simulink model "detumbling"  (R2023b)
settings: Solver=VariableStepAuto  StartTime=0.0  StopTime=10.0  RelTol=1e-3
values from neighbouring files (symbols this model uses):
  ARW = deg2rad(0.10)    [main_group24.m]
  Cd = 2.2    [main_group24.m]
  GyroSampleRate = 10    [main_group24.m]
  Ix = J(1,1)    [Air_Drag_script.m]    (also in data_mass.m = 0.0755003333333; main.m = 0.057749855; main_group24.m = 0.0755003333333)
  Iy = J(2,2)    [Air_Drag_script.m]    (also in data_mass.m = 0.0755003333333; main.m = 0.04143542; main_group24.m = 0.0755003333333)
  Iz = J(3,3)    [Air_Drag_script.m]    (also in data_mass.m = 0.055; main.m = 0.024624309; main_group24.m = 0.055)
  J = diag([100.9 25.1 91.6])*1e-2    [Air_Drag_script.m]
  MMnoise = 15e-9*[1; 1; 1]    [main_group24.m]
  MMSampleRate = 1    [main_group24.m]
  P = Fe/c    (= 4.52980041279e-06)    [main_group24.m]
  rho_air = 1.65e-13    [Air_Drag_script.m]    (also in main_group24.m = 6.967e-13)
  rho_d_body = 0.1*2/3    (= 0.0666666666667)    [main_group24.m]
  rho_d_sp = 0.1*2/3    (= 0.0666666666667)    [main_group24.m]
  rho_s_body = 0.5    [main_group24.m]
  rho_s_sp = 0.1    [main_group24.m]
  RRW = deg2rad(0.3)    [main_group24.m]
undefined symbols (not defined in the file or in its folder): invJ, omega_0b, pan1, pan2, s1, s2, s3, s4, s5, s6, v_rel
libraries: vrlib x21, sharedutil x2
settings Model: Creator=hp  LastModifiedBy=hp

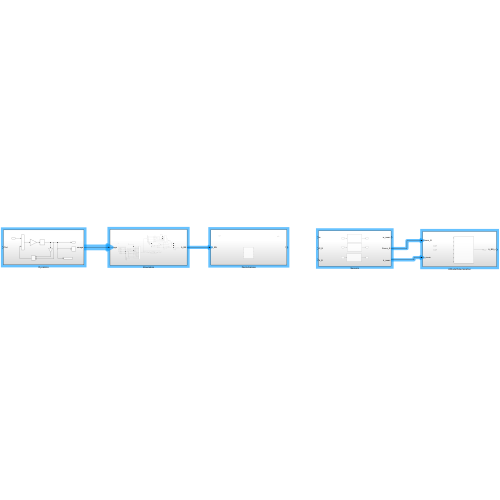
[thumbnail: Simulink's stored preview of the top-level diagram]
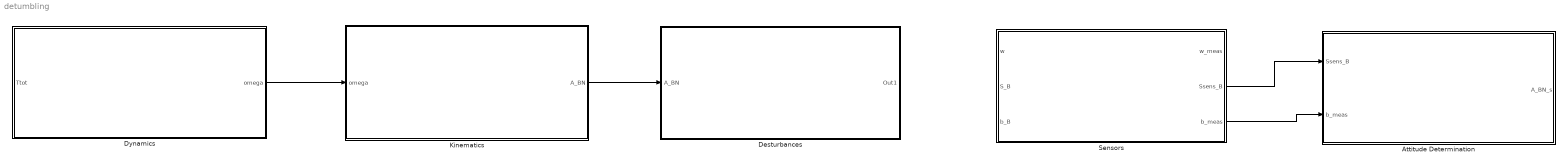
== system detumbling ==
  Attitude Determination : Subsystem
  Desturbances : Subsystem
  Dynamics : Subsystem
  Kinematics : Subsystem
  Sensors : Subsystem
  wires:
  Sensors/3(b_meas) -> Attitude Determination/2(b_meas)
  Kinematics/1(A_BN) -> Desturbances/1(A_BN)
  Sensors/2(Ssens_B) -> Attitude Determination/1(Ssens_B)
  Dynamics/1(omega) -> Kinematics/1(omega)

== system detumbling/Attitude Determination ==
  Ssens_B : Inport
  b_meas : Inport  Port=2
  Attitude Determination : MATLAB Function  TreatAsAtomicUnit=on
  A_BN_s : Outport
  wires:
  Attitude Determination/1(A_BN_s) -> A_BN_s/1  "A_BN_s"

== system detumbling/Desturbances ==
  A_BN : Inport
  Disturbance : Subsystem
  Out1 : Outport

== system detumbling/Dynamics ==
  note: omega
  Ttot : Inport
  Add : Sum
  Cross Product : vrlib/Utilities/Cross Product
  Gain : Gain  Gain=invJ  Multiplication=Matrix(K*u)
  Gain1 : Gain  Gain=J  Multiplication=Matrix(K*u)
  Integrator3 : Integrator  InitialCondition=omega_0b  AbsoluteTolerance=10^-7
  Scope : Scope
  To Workspace : ToWorkspace  VariableName=det  SaveFormat=Timeseries  SampleTime=-1
  omega : Outport
  wires:
  Gain1/1 -> Cross Product/1
  Ttot/1 -> Add/1
  Cross Product/1 -> Add/2
  Integrator3/1 -> To Workspace/1, Scope/1, omega/1, Cross Product/2, Gain1/1
  Gain/1 -> Integrator3/1
  Add/1 -> Gain/1

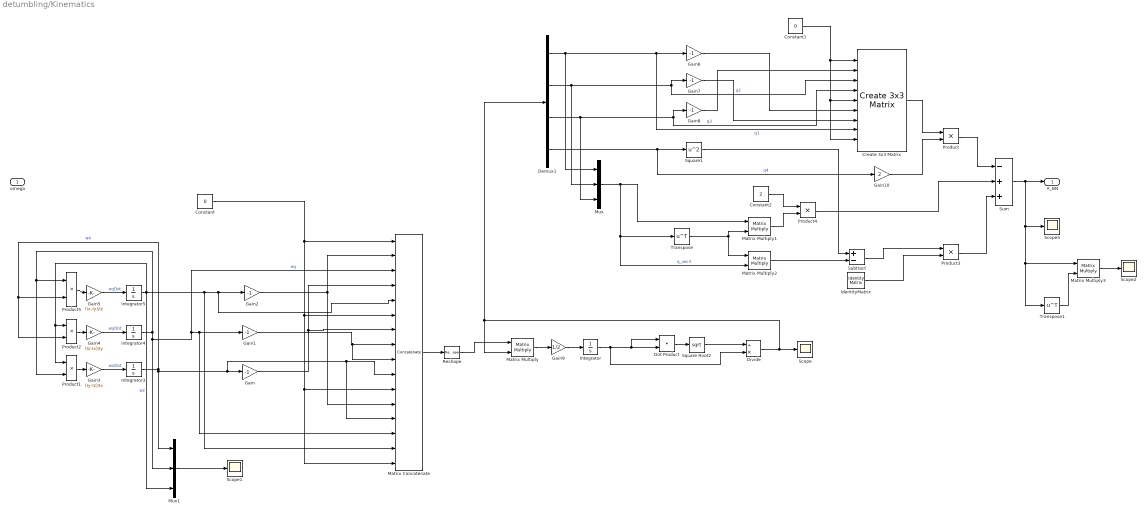
== system detumbling/Kinematics ==
  omega : Inport
  Constant : Constant  Value=0
  Constant1 : Constant  Value=0
  Constant2 : Constant  Value=2
  Create 3x3 Matrix : sharedutil/Create 3x3 Matrix  aMode=aMode
      settings: LibrarySourceBlock=aerolibutil/Create 3x3 Matrix
  Demux1 : Demux
  Divide : Product  Inputs=/*
  Dot Product : DotProduct  OutDataTypeStr=Inherit: Inherit via internal rule
  Gain{,1..2,6..8} (6 alike) : Gain  Gain=-1
  Gain10 : Gain  Gain=2
  Gain3 : Gain  Gain=(Iy-Iz)/Ix
  Gain4 : Gain  Gain=(Iz-Ix)/Iy
  Gain5 : Gain  Gain=(Ix-Iy)/Iz
  Gain9 : Gain  Gain=1/2
  IdentityMatrix : IdentityMatrix  OutputDimensions=3
  Integrator : Integrator  InitialCondition=[0 0 0 1]
  Integrator3 : Integrator  InitialCondition=omega_0b(1)
  Integrator4 : Integrator  InitialCondition=omega_0b(2)
  Integrator5 : Integrator  InitialCondition=omega_0b(3)
  Matrix Concatenate : Concatenate  NumInputs=16  Mode=Multidimensional array  ConcatenateDimension=2
  Matrix Multiply{,1..3} (4 alike) : Product  Multiplication=Matrix(*)
  Mux : Mux  Inputs=3
  Mux1 : Mux  Inputs=3
  Product{,1..5} (6 alike) : Product
  Reshape : Reshape  OutputDimensionality=Customize  OutputDimensions=[4,4]
  Scope{,1..2,5} (4 alike) : Scope
  Square Root2 : Sqrt
  Square1 : Math  Operator=square
  Subtract : Sum  Inputs=+-
  Sum : Sum  Inputs=-++
  Transpose : Math  Operator=transpose
  Transpose1 : Math  Operator=transpose
  A_BN : Outport
  wires:
  Matrix Multiply/1 -> Gain9/1
  Square Root2/1 -> Divide/1
  Product1/1 -> Gain3/1
  Gain1/1 -> Matrix Concatenate/9, Matrix Concatenate/8
  Product5/1 -> Gain5/1
  Constant/1 -> Matrix Concatenate/16, Matrix Concatenate/11, Matrix Concatenate/6, Matrix Concatenate/1
  Gain3/1 -> Integrator3/1  "wxDot"
  Gain/1 -> Matrix Concatenate/7, Matrix Concatenate/4
  Integrator/1 -> Dot Product/1, Dot Product/2, Divide/2
  Matrix Concatenate/1 -> Reshape/1
  Integrator5/1 -> Mux1/3, Matrix Concatenate/15, Matrix Concatenate/5, Gain2/1, Product1/1, Product2/1  "wz"
  Gain4/1 -> Integrator4/1  "wyDot"
  Gain2/1 -> Matrix Concatenate/12, Matrix Concatenate/2
  Gain5/1 -> Integrator5/1  "wzDot"
  Integrator4/1 -> Matrix Concatenate/3, Matrix Concatenate/14, Gain1/1, Mux1/2, Product1/2, Product5/1  "wy"
  Integrator3/1 -> Matrix Concatenate/13, Matrix Concatenate/10, Gain/1, Mux1/1, Product2/2, Product5/2  "wx"
  Product2/1 -> Gain4/1
  Constant1/1 -> Create 3x3 Matrix/5, Create 3x3 Matrix/9, Create 3x3 Matrix/1
  Demux1/1 -> Mux/1, Gain6/1, Create 3x3 Matrix/8  "q1"
  Demux1/2 -> Mux/2, Gain7/1, Create 3x3 Matrix/3  "q2"
  Demux1/4 -> Gain10/1, Square1/1  "q4"
  Gain8/1 -> Create 3x3 Matrix/2
  Gain6/1 -> Create 3x3 Matrix/6
  Gain7/1 -> Create 3x3 Matrix/7
  Transpose/1 -> Matrix Multiply1/2, Matrix Multiply2/1
  Gain10/1 -> Product/2
  Create 3x3 Matrix/1 -> Product/1
  Square1/1 -> Subtract/1
  Matrix Multiply2/1 -> Subtract/2
  Divide/1 -> Scope/1, Demux1/1, Matrix Multiply/2
  Subtract/1 -> Product3/1
  IdentityMatrix/1 -> Product3/2
  Product/1 -> Sum/1
  Product3/1 -> Sum/3
  Constant2/1 -> Product4/1
  Matrix Multiply1/1 -> Product4/2
  Product4/1 -> Sum/2
  Demux1/3 -> Mux/3, Gain8/1, Create 3x3 Matrix/4  "q3"
  Mux/1 -> Matrix Multiply1/1, Transpose/1, Matrix Multiply2/2  "q_vec3"
  Mux1/1 -> Scope1/1
  Sum/1 -> Transpose1/1, Matrix Multiply3/1, Scope5/1, A_BN/1
  Transpose1/1 -> Matrix Multiply3/2
  Matrix Multiply3/1 -> Scope2/1
  Dot Product/1 -> Square Root2/1
  Reshape/1 -> Matrix Multiply/1
  Gain9/1 -> Integrator/1

== system detumbling/Sensors ==
  w : Inport
  S_B : Inport  Port=2
  b_B : Inport  Port=3
  Gyroscope : Subsystem
  Magnetometer : Subsystem
  Sun Sensor : Subsystem
  w_meas : Outport
  Ssens_B : Outport  Port=2
  b_meas : Outport  Port=3
  wires:
  w/1 -> Gyroscope/1(w)
  Gyroscope/1(w_meas) -> w_meas/1
  Sun Sensor/1(Ssens_B) -> Ssens_B/1
  S_B/1 -> Sun Sensor/1(S_B)
  b_B/1 -> Magnetometer/1(b_B)
  Magnetometer/1(MM_meas) -> b_meas/1

== system detumbling/Desturbances/Disturbance ==
  r_s_B : Inport
  v_rel_B : Inport  Port=2
  In4 : Inport  Port=3
  Air Drag : Subsystem
  Gravity Gradient : Subsystem
  Magnetic Field : Subsystem
  Solar Rsdiation Pressure : Subsystem
  Tsrp : Outport
  Tair : Outport  Port=2
  Out3 : Outport  Port=3
  Out4 : Outport  Port=4
  wires:
  r_s_B/1 -> Solar Rsdiation Pressure/1(r_s_B)
  In4/1 -> Magnetic Field/1(In1)
  Air Drag/1(Tair) -> Tair/1
  v_rel_B/1 -> Air Drag/1(v_rel_B)
  Magnetic Field/1(Out1) -> Out4/1
  Solar Rsdiation Pressure/1(Tsrp) -> Tsrp/1
  Gravity Gradient/1(Out1) -> Out3/1

== system detumbling/Sensors/Gyroscope ==
  note: w_BN_measured = G(w_B) A_eps w_BN + n + b
  w : Inport
  ARW : RandomNumber  Variance=(deg2rad(ARW)/sqrt(3600)/sqrt(1/GyroSampleRate))^2*[1;1;1]  SampleTime=1/GyroSampleRate
  Integrator : Integrator
  RRW : RandomNumber  Variance=(deg2rad(RRW)/3600/sqrt(1/GyroSampleRate))^2* [1;1;1]  SampleTime=1/GyroSampleRate
  Sensor Sampling frequency : ZeroOrderHold  SampleTime=-1
  Sum : Sum  Inputs=+++
  w_meas : Outport
  wires:
  RRW/1 -> Integrator/1  "b_dot"
  ARW/1 -> Sum/2  "n"
  Integrator/1 -> Sum/3  "b"
  w/1 -> Sensor Sampling frequency/1
  Sum/1 -> w_meas/1
  Sensor Sampling frequency/1 -> Sum/1

== system detumbling/Sensors/Magnetometer ==
  b_B : Inport
  Constant : Constant  Value=MMnoise
  MatrixMultiply : Product  Multiplication=Matrix(*)
  Subsystem : Subsystem
  Sum : Sum
  MM_meas : Outport
  wires:
  Constant/1 -> Sum/2
  b_B/1 -> Sum/1  "b_B"
  Subsystem/1(A_epsMM) -> MatrixMultiply/1
  Sum/1 -> MatrixMultiply/2
  MatrixMultiply/1 -> MM_meas/1

== system detumbling/Sensors/Sun Sensor ==
  S_B : Inport
  Matrix Multiply1 : Product  Multiplication=Matrix(*)
  Subsystem : Subsystem
  Ssens_B : Outport
  wires:
  S_B/1 -> Matrix Multiply1/2
  Subsystem/1(A_eps) -> Matrix Multiply1/1  "A_eps"
  Matrix Multiply1/1 -> Ssens_B/1

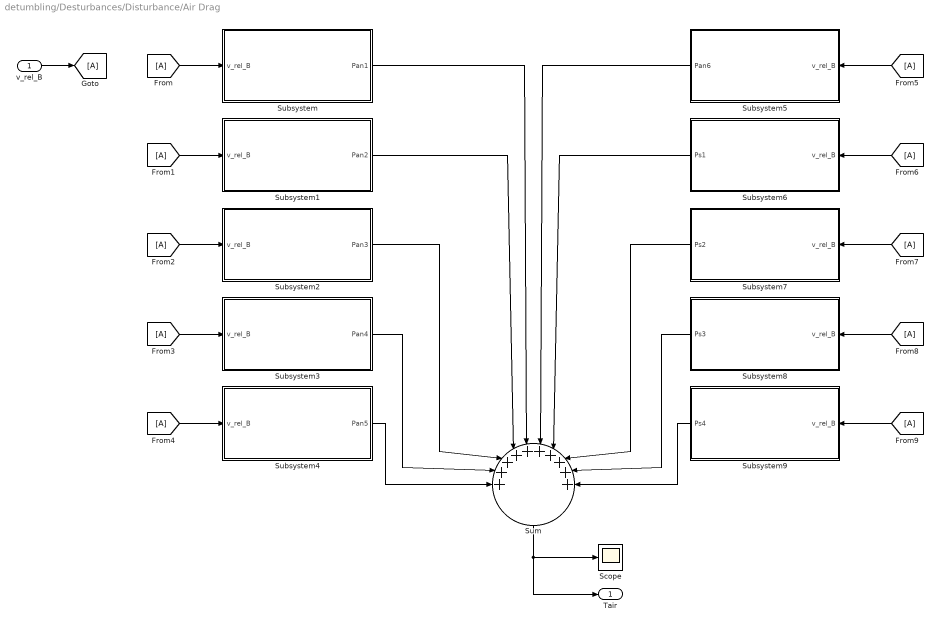
== system detumbling/Desturbances/Disturbance/Air Drag ==
  v_rel_B : Inport
  From{,1..9} (10 alike) : From
  Goto : Goto
  Scope : Scope
  Subsystem : Subsystem
  Subsystem1 : Subsystem
  Subsystem2 : Subsystem
  Subsystem3 : Subsystem
  Subsystem4 : Subsystem
  Subsystem5 : Subsystem
  Subsystem6 : Subsystem
  Subsystem7 : Subsystem
  Subsystem8 : Subsystem
  Subsystem9 : Subsystem
  Sum : Sum  Inputs=++++++++++
  Tair : Outport
  wires:
  Sum/1 -> Scope/1, Tair/1
  v_rel_B/1 -> Goto/1
  From5/1 -> Subsystem5/1(v_rel_B)
  From6/1 -> Subsystem6/1(v_rel_B)
  From7/1 -> Subsystem7/1(v_rel_B)
  From8/1 -> Subsystem8/1(v_rel_B)
  From9/1 -> Subsystem9/1(v_rel_B)
  From4/1 -> Subsystem4/1(v_rel_B)
  From3/1 -> Subsystem3/1(v_rel_B)
  From2/1 -> Subsystem2/1(v_rel_B)
  From1/1 -> Subsystem1/1(v_rel_B)
  From/1 -> Subsystem/1(v_rel_B)
  Subsystem4/1(Pan5) -> Sum/1
  Subsystem3/1(Pan4) -> Sum/2
  Subsystem2/1(Pan3) -> Sum/3
  Subsystem1/1(Pan2) -> Sum/4
  Subsystem/1(Pan1) -> Sum/5
  Subsystem5/1(Pan6) -> Sum/6
  Subsystem6/1(Ps1) -> Sum/7
  Subsystem7/1(Ps2) -> Sum/8
  Subsystem8/1(Ps3) -> Sum/9
  Subsystem9/1(Ps4) -> Sum/10

== system detumbling/Desturbances/Disturbance/Gravity Gradient ==
  Constant : Constant
  Out1 : Outport

== system detumbling/Desturbances/Disturbance/Magnetic Field ==
  In1 : Inport
  Out1 : Outport
  wires:
  In1/1 -> Out1/1

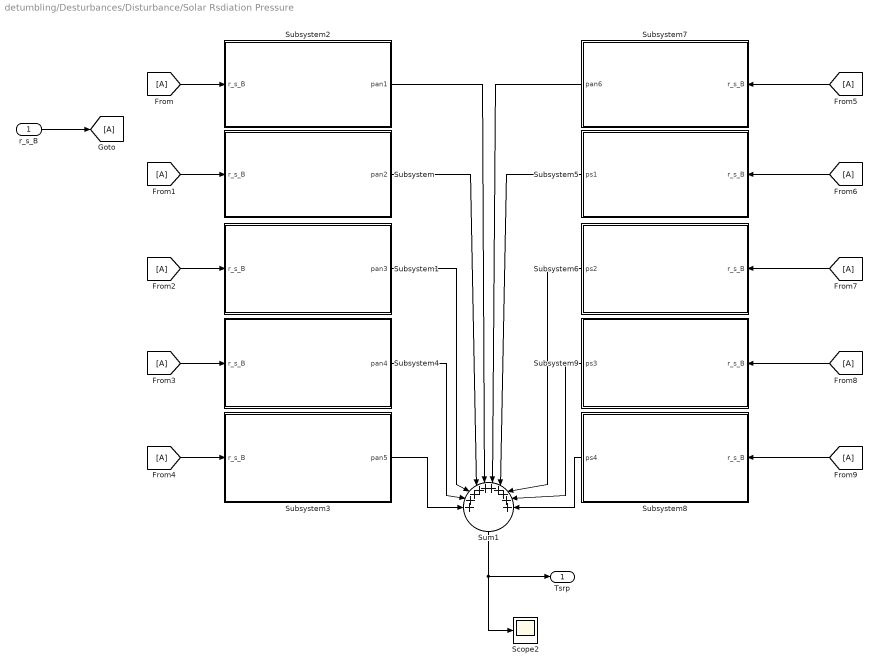
== system detumbling/Desturbances/Disturbance/Solar Rsdiation Pressure ==
  r_s_B : Inport
  From{,1..9} (10 alike) : From
  Goto : Goto
  Scope2 : Scope
  Subsystem : Subsystem
  Subsystem1 : Subsystem
  Subsystem2 : Subsystem
  Subsystem3 : Subsystem
  Subsystem4 : Subsystem
  Subsystem5 : Subsystem
  Subsystem6 : Subsystem
  Subsystem7 : Subsystem
  Subsystem8 : Subsystem
  Subsystem9 : Subsystem
  Sum1 : Sum  Inputs=++++++++++
  Tsrp : Outport
  wires:
  r_s_B/1 -> Goto/1
  Sum1/1 -> Tsrp/1, Scope2/1
  Subsystem7/1(pan6) -> Sum1/6
  From1/1 -> Subsystem/1(r_s_B)
  From8/1 -> Subsystem9/1(r_s_B)
  Subsystem1/1(pan3) -> Sum1/3
  Subsystem/1(pan2) -> Sum1/4
  From/1 -> Subsystem2/1(r_s_B)
  Subsystem2/1(pan1) -> Sum1/5
  Subsystem4/1(pan4) -> Sum1/2
  Subsystem9/1(ps3) -> Sum1/9
  From9/1 -> Subsystem8/1(r_s_B)
  Subsystem8/1(ps4) -> Sum1/10
  Subsystem3/1(pan5) -> Sum1/1
  From7/1 -> Subsystem6/1(r_s_B)
  Subsystem5/1(ps1) -> Sum1/7
  From3/1 -> Subsystem4/1(r_s_B)
  From5/1 -> Subsystem7/1(r_s_B)
  From6/1 -> Subsystem5/1(r_s_B)
  From2/1 -> Subsystem1/1(r_s_B)
  Subsystem6/1(ps2) -> Sum1/8
  From4/1 -> Subsystem3/1(r_s_B)

== system detumbling/Sensors/Magnetometer/Subsystem ==
  Constant : Constant
  Display : Display
  Gain : Gain  Gain=[1; -1; 1]
  Gain1 : Gain  Gain=[1; 1; -1]
  Gain2 : Gain  Gain=[-1; 1; 1]
  Matrix Concatenate : Concatenate  NumInputs=3  Mode=Multidimensional array  ConcatenateDimension=2
  Random Number : RandomNumber  Variance=deg2rad(0.1)^2  Seed=5  SampleTime=1/MMSampleRate
  Random Number1 : RandomNumber  Variance=deg2rad(0.1)^2  Seed=6  SampleTime=1/MMSampleRate
  Random Number2 : RandomNumber  Variance=deg2rad(0.1)^2  Seed=7  SampleTime=1/MMSampleRate
  Selector : Selector  InputPortWidth=4  IndexOptions=Index vector (dialog)  Indices=[1 4 3]  OutputSizes=1
  Selector1 : Selector  InputPortWidth=4  IndexOptions=Index vector (dialog)  Indices=[4 1 2]  OutputSizes=1
  Selector2 : Selector  InputPortWidth=4  IndexOptions=Index vector (dialog)  Indices=[3 2 1]  OutputSizes=1
  Vector Concatenate : Concatenate  NumInputs=4
  A_epsMM : Outport
  wires:
  Selector2/1 -> Gain2/1
  Selector/1 -> Gain/1
  Gain/1 -> Matrix Concatenate/1
  Random Number/1 -> Vector Concatenate/2
  Matrix Concatenate/1 -> Display/1, A_epsMM/1
  Selector1/1 -> Gain1/1
  Vector Concatenate/1 -> Selector2/1, Selector/1, Selector1/1
  Gain2/1 -> Matrix Concatenate/3
  Constant/1 -> Vector Concatenate/1
  Gain1/1 -> Matrix Concatenate/2
  Random Number2/1 -> Vector Concatenate/4
  Random Number1/1 -> Vector Concatenate/3

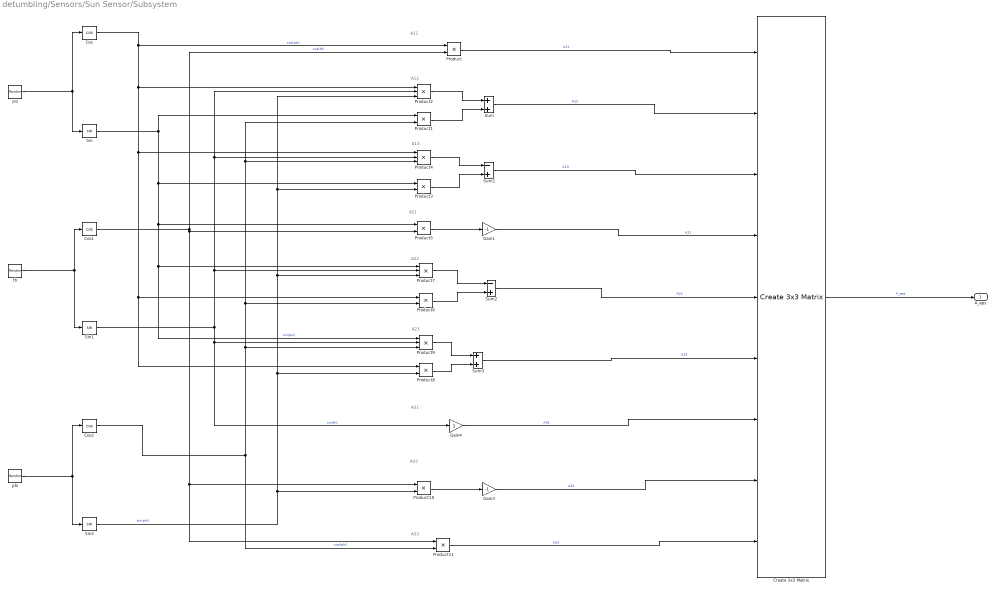
== system detumbling/Sensors/Sun Sensor/Subsystem ==
  note: A31
  note: A33
  note: A32
  note: A23
  note: A22
  note: A21
  note: A13
  note: A12
  note: A11
  Cos : Trigonometry  Operator=cos
  Cos1 : Trigonometry  Operator=cos
  Cos2 : Trigonometry  Operator=cos
  Create 3x3 Matrix : sharedutil/Create 3x3 Matrix  aMode=aMode
  Gain1 : Gain  Gain=-1
  Gain3 : Gain  Gain=-1
  Gain4 : Gain
  Product{,1,3,5..6,8,10..11} (8 alike) : Product
  Product{2,4,7,9} (4 alike) : Product  Inputs=3
  Sin : Trigonometry
  Sin1 : Trigonometry
  Sin2 : Trigonometry
  Sum : Sum
  Sum1 : Sum  Inputs=-+
  Sum2 : Sum  Inputs=-+
  Sum3 : Sum
  phi : RandomNumber  Variance=(1/8*pi/180)^2  Seed=2  SampleTime=0.2
  psi : RandomNumber  Variance=(1/8*pi/180)^2  SampleTime=0.2
  th : RandomNumber  Variance=(1/8*pi/180)^2  Seed=1  SampleTime=0.2
  A_eps : Outport
  wires:
  psi/1 -> Cos/1, Sin/1
  th/1 -> Sin1/1, Cos1/1
  phi/1 -> Sin2/1, Cos2/1
  Product2/1 -> Sum/1
  Product1/1 -> Sum/2
  Product3/1 -> Sum1/2
  Product4/1 -> Sum1/1
  Product7/1 -> Sum2/1
  Product6/1 -> Sum2/2
  Product9/1 -> Sum3/1
  Product8/1 -> Sum3/2
  Gain4/1 -> Create 3x3 Matrix/7  "A31"
  Product/1 -> Create 3x3 Matrix/1  "A11"
  Sum/1 -> Create 3x3 Matrix/2  "A12"
  Sum1/1 -> Create 3x3 Matrix/3  "A13"
  Product5/1 -> Gain1/1
  Sum2/1 -> Create 3x3 Matrix/5  "A22"
  Sum3/1 -> Create 3x3 Matrix/6  "A23"
  Product10/1 -> Gain3/1
  Product11/1 -> Create 3x3 Matrix/9  "A33"
  Gain1/1 -> Create 3x3 Matrix/4  "A21"
  Gain3/1 -> Create 3x3 Matrix/8  "A32"
  Cos/1 -> Product8/1, Product6/1, Product4/1, Product2/1, Product/1  "cos(psi)"
  Cos1/1 -> Product/2, Product11/1, Product10/1, Product5/2  "cos(th)"
  Sin1/1 -> Gain4/1, Product9/2, Product7/2, Product2/2, Product4/2  "sin(th)"
  Sin2/1 -> Product7/3, Product3/2, Product2/3, Product8/2, Product10/2  "sin(phi)"
  Sin/1 -> Product3/1, Product5/1, Product7/1, Product9/1, Product1/1  "sin(psi)"
  Cos2/1 -> Product6/2, Product4/3, Product1/2, Product9/3, Product11/2  "cos(phi)"
  Create 3x3 Matrix/1 -> A_eps/1  "A_eps"

== system detumbling/Desturbances/Disturbance/Air Drag/Subsystem ==
  v_rel_B : Inport
  Constant : Constant  Value=-0.5
  Constant1 : Constant  Value=s1.n
  Constant2 : Constant  Value=s1.r
  Constant3 : Constant  Value=s1.A
  Cross Product2 : vrlib/Utilities/Cross Product
  Dot Product1 : DotProduct  OutDataTypeStr=Inherit: Inherit via internal rule
  Gain : Gain  Gain=rho_air
  Gain1 : Gain  Gain=0
  Gain2 : Gain  Gain=Cd
  Gain3 : Gain  Gain=v_rel^2
  Product : Product  Inputs=4
  Switch1 : Switch  Criteria=u2 > Threshold  SaturateOnIntegerOverflow=off  InputSameDT=off
  Pan1 : Outport
  wires:
  Constant2/1 -> Cross Product2/1
  Gain1/1 -> Switch1/3
  Dot Product1/1 -> Gain1/1, Switch1/2, Switch1/1
  Constant3/1 -> Product/2
  Product/1 -> Cross Product2/2
  Switch1/1 -> Product/4
  v_rel_B/1 -> Dot Product1/1, Product/3
  Gain3/1 -> Product/1
  Gain/1 -> Gain2/1
  Constant/1 -> Gain/1
  Cross Product2/1 -> Pan1/1
  Constant1/1 -> Dot Product1/2
  Gain2/1 -> Gain3/1

== system detumbling/Desturbances/Disturbance/Air Drag/Subsystem1 ==
  v_rel_B : Inport
  Constant : Constant  Value=-0.5
  Constant1 : Constant  Value=s1.n
  Constant2 : Constant  Value=s1.r
  Constant3 : Constant  Value=s1.A
  Cross Product2 : vrlib/Utilities/Cross Product
  Dot Product1 : DotProduct  OutDataTypeStr=Inherit: Inherit via internal rule
  Gain : Gain  Gain=rho_air
  Gain1 : Gain  Gain=0
  Gain2 : Gain  Gain=Cd
  Gain3 : Gain  Gain=v_rel^2
  Product : Product  Inputs=4
  Switch1 : Switch  Criteria=u2 > Threshold  SaturateOnIntegerOverflow=off  InputSameDT=off
  Pan2 : Outport
  wires:
  Gain2/1 -> Gain3/1
  Constant1/1 -> Dot Product1/2
  Cross Product2/1 -> Pan2/1
  Constant/1 -> Gain/1
  Gain/1 -> Gain2/1
  Gain3/1 -> Product/1
  v_rel_B/1 -> Product/3, Dot Product1/1
  Switch1/1 -> Product/4
  Product/1 -> Cross Product2/2
  Constant3/1 -> Product/2
  Dot Product1/1 -> Switch1/1, Switch1/2, Gain1/1
  Gain1/1 -> Switch1/3
  Constant2/1 -> Cross Product2/1

== system detumbling/Desturbances/Disturbance/Air Drag/Subsystem2 ==
  v_rel_B : Inport
  Constant : Constant  Value=-0.5
  Constant1 : Constant  Value=s1.n
  Constant2 : Constant  Value=s1.r
  Constant3 : Constant  Value=s1.A
  Cross Product2 : vrlib/Utilities/Cross Product
  Dot Product1 : DotProduct  OutDataTypeStr=Inherit: Inherit via internal rule
  Gain : Gain  Gain=rho_air
  Gain1 : Gain  Gain=0
  Gain2 : Gain  Gain=Cd
  Gain3 : Gain  Gain=v_rel^2
  Product : Product  Inputs=4
  Switch1 : Switch  Criteria=u2 > Threshold  SaturateOnIntegerOverflow=off  InputSameDT=off
  Pan3 : Outport
  wires:
  Constant2/1 -> Cross Product2/1
  Gain1/1 -> Switch1/3
  Dot Product1/1 -> Gain1/1, Switch1/2, Switch1/1
  Constant3/1 -> Product/2
  Product/1 -> Cross Product2/2
  Switch1/1 -> Product/4
  v_rel_B/1 -> Dot Product1/1, Product/3
  Gain3/1 -> Product/1
  Gain/1 -> Gain2/1
  Constant/1 -> Gain/1
  Cross Product2/1 -> Pan3/1
  Constant1/1 -> Dot Product1/2
  Gain2/1 -> Gain3/1

== system detumbling/Desturbances/Disturbance/Air Drag/Subsystem3 ==
  v_rel_B : Inport
  Constant : Constant  Value=-0.5
  Constant1 : Constant  Value=s1.n
  Constant2 : Constant  Value=s1.r
  Constant3 : Constant  Value=s1.A
  Cross Product2 : vrlib/Utilities/Cross Product
  Dot Product1 : DotProduct  OutDataTypeStr=Inherit: Inherit via internal rule
  Gain : Gain  Gain=rho_air
  Gain1 : Gain  Gain=0
  Gain2 : Gain  Gain=Cd
  Gain3 : Gain  Gain=v_rel^2
  Product : Product  Inputs=4
  Switch1 : Switch  Criteria=u2 > Threshold  SaturateOnIntegerOverflow=off  InputSameDT=off
  Pan4 : Outport
  wires:
  Gain2/1 -> Gain3/1
  Constant1/1 -> Dot Product1/2
  Cross Product2/1 -> Pan4/1
  Constant/1 -> Gain/1
  Gain/1 -> Gain2/1
  Gain3/1 -> Product/1
  v_rel_B/1 -> Product/3, Dot Product1/1
  Switch1/1 -> Product/4
  Product/1 -> Cross Product2/2
  Constant3/1 -> Product/2
  Dot Product1/1 -> Switch1/1, Switch1/2, Gain1/1
  Gain1/1 -> Switch1/3
  Constant2/1 -> Cross Product2/1

== system detumbling/Desturbances/Disturbance/Air Drag/Subsystem4 ==
  v_rel_B : Inport
  Constant : Constant  Value=-0.5
  Constant1 : Constant  Value=s1.n
  Constant2 : Constant  Value=s1.r
  Constant3 : Constant  Value=s1.A
  Cross Product2 : vrlib/Utilities/Cross Product
  Dot Product1 : DotProduct  OutDataTypeStr=Inherit: Inherit via internal rule
  Gain : Gain  Gain=rho_air
  Gain1 : Gain  Gain=0
  Gain2 : Gain  Gain=Cd
  Gain3 : Gain  Gain=v_rel^2
  Product : Product  Inputs=4
  Switch1 : Switch  Criteria=u2 > Threshold  SaturateOnIntegerOverflow=off  InputSameDT=off
  Pan5 : Outport
  wires:
  Constant2/1 -> Cross Product2/1
  Gain1/1 -> Switch1/3
  Dot Product1/1 -> Gain1/1, Switch1/2, Switch1/1
  Constant3/1 -> Product/2
  Product/1 -> Cross Product2/2
  Switch1/1 -> Product/4
  v_rel_B/1 -> Dot Product1/1, Product/3
  Gain3/1 -> Product/1
  Gain/1 -> Gain2/1
  Constant/1 -> Gain/1
  Cross Product2/1 -> Pan5/1
  Constant1/1 -> Dot Product1/2
  Gain2/1 -> Gain3/1

== system detumbling/Desturbances/Disturbance/Air Drag/Subsystem5 ==
  v_rel_B : Inport
  Constant : Constant  Value=-0.5
  Constant1 : Constant  Value=s1.n
  Constant2 : Constant  Value=s1.r
  Constant3 : Constant  Value=s1.A
  Cross Product2 : vrlib/Utilities/Cross Product
  Dot Product1 : DotProduct  OutDataTypeStr=Inherit: Inherit via internal rule
  Gain : Gain  Gain=rho_air
  Gain1 : Gain  Gain=0
  Gain2 : Gain  Gain=Cd
  Gain3 : Gain  Gain=v_rel^2
  Product : Product  Inputs=4
  Switch1 : Switch  Criteria=u2 > Threshold  SaturateOnIntegerOverflow=off  InputSameDT=off
  Pan6 : Outport
  wires:
  Constant2/1 -> Cross Product2/1
  Gain1/1 -> Switch1/3
  Dot Product1/1 -> Gain1/1, Switch1/2, Switch1/1
  Constant3/1 -> Product/2
  Product/1 -> Cross Product2/2
  Switch1/1 -> Product/4
  v_rel_B/1 -> Dot Product1/1, Product/3
  Gain3/1 -> Product/1
  Gain/1 -> Gain2/1
  Constant/1 -> Gain/1
  Cross Product2/1 -> Pan6/1
  Constant1/1 -> Dot Product1/2
  Gain2/1 -> Gain3/1

== system detumbling/Desturbances/Disturbance/Air Drag/Subsystem6 ==
  v_rel_B : Inport
  Constant : Constant  Value=-0.5
  Constant1 : Constant  Value=s1.n
  Constant2 : Constant  Value=s1.r
  Constant3 : Constant  Value=s1.A
  Cross Product2 : vrlib/Utilities/Cross Product
  Dot Product1 : DotProduct  OutDataTypeStr=Inherit: Inherit via internal rule
  Gain : Gain  Gain=rho_air
  Gain1 : Gain  Gain=0
  Gain2 : Gain  Gain=Cd
  Gain3 : Gain  Gain=v_rel^2
  Product : Product  Inputs=4
  Switch1 : Switch  Criteria=u2 > Threshold  SaturateOnIntegerOverflow=off  InputSameDT=off
  Ps1 : Outport
  wires:
  Gain2/1 -> Gain3/1
  Constant1/1 -> Dot Product1/2
  Cross Product2/1 -> Ps1/1
  Constant/1 -> Gain/1
  Gain/1 -> Gain2/1
  Gain3/1 -> Product/1
  v_rel_B/1 -> Product/3, Dot Product1/1
  Switch1/1 -> Product/4
  Product/1 -> Cross Product2/2
  Constant3/1 -> Product/2
  Dot Product1/1 -> Switch1/1, Switch1/2, Gain1/1
  Gain1/1 -> Switch1/3
  Constant2/1 -> Cross Product2/1

== system detumbling/Desturbances/Disturbance/Air Drag/Subsystem7 ==
  v_rel_B : Inport
  Constant : Constant  Value=-0.5
  Constant1 : Constant  Value=s1.n
  Constant2 : Constant  Value=s1.r
  Constant3 : Constant  Value=s1.A
  Cross Product2 : vrlib/Utilities/Cross Product
  Dot Product1 : DotProduct  OutDataTypeStr=Inherit: Inherit via internal rule
  Gain : Gain  Gain=rho_air
  Gain1 : Gain  Gain=0
  Gain2 : Gain  Gain=Cd
  Gain3 : Gain  Gain=v_rel^2
  Product : Product  Inputs=4
  Switch1 : Switch  Criteria=u2 > Threshold  SaturateOnIntegerOverflow=off  InputSameDT=off
  Ps2 : Outport
  wires:
  Constant2/1 -> Cross Product2/1
  Gain1/1 -> Switch1/3
  Dot Product1/1 -> Gain1/1, Switch1/2, Switch1/1
  Constant3/1 -> Product/2
  Product/1 -> Cross Product2/2
  Switch1/1 -> Product/4
  v_rel_B/1 -> Dot Product1/1, Product/3
  Gain3/1 -> Product/1
  Gain/1 -> Gain2/1
  Constant/1 -> Gain/1
  Cross Product2/1 -> Ps2/1
  Constant1/1 -> Dot Product1/2
  Gain2/1 -> Gain3/1

== system detumbling/Desturbances/Disturbance/Air Drag/Subsystem8 ==
  v_rel_B : Inport
  Constant : Constant  Value=-0.5
  Constant1 : Constant  Value=s1.n
  Constant2 : Constant  Value=s1.r
  Constant3 : Constant  Value=s1.A
  Cross Product2 : vrlib/Utilities/Cross Product
  Dot Product1 : DotProduct  OutDataTypeStr=Inherit: Inherit via internal rule
  Gain : Gain  Gain=rho_air
  Gain1 : Gain  Gain=0
  Gain2 : Gain  Gain=Cd
  Gain3 : Gain  Gain=v_rel^2
  Product : Product  Inputs=4
  Switch1 : Switch  Criteria=u2 > Threshold  SaturateOnIntegerOverflow=off  InputSameDT=off
  Ps3 : Outport
  wires:
  Gain2/1 -> Gain3/1
  Constant1/1 -> Dot Product1/2
  Cross Product2/1 -> Ps3/1
  Constant/1 -> Gain/1
  Gain/1 -> Gain2/1
  Gain3/1 -> Product/1
  v_rel_B/1 -> Product/3, Dot Product1/1
  Switch1/1 -> Product/4
  Product/1 -> Cross Product2/2
  Constant3/1 -> Product/2
  Dot Product1/1 -> Switch1/1, Switch1/2, Gain1/1
  Gain1/1 -> Switch1/3
  Constant2/1 -> Cross Product2/1

== system detumbling/Desturbances/Disturbance/Air Drag/Subsystem9 ==
  v_rel_B : Inport
  Constant : Constant  Value=-0.5
  Constant1 : Constant  Value=s1.n
  Constant2 : Constant  Value=s1.r
  Constant3 : Constant  Value=s1.A
  Cross Product2 : vrlib/Utilities/Cross Product
  Dot Product1 : DotProduct  OutDataTypeStr=Inherit: Inherit via internal rule
  Gain : Gain  Gain=rho_air
  Gain1 : Gain  Gain=0
  Gain2 : Gain  Gain=Cd
  Gain3 : Gain  Gain=v_rel^2
  Product : Product  Inputs=4
  Switch1 : Switch  Criteria=u2 > Threshold  SaturateOnIntegerOverflow=off  InputSameDT=off
  Ps4 : Outport
  wires:
  Constant2/1 -> Cross Product2/1
  Gain1/1 -> Switch1/3
  Dot Product1/1 -> Gain1/1, Switch1/2, Switch1/1
  Constant3/1 -> Product/2
  Product/1 -> Cross Product2/2
  Switch1/1 -> Product/4
  v_rel_B/1 -> Dot Product1/1, Product/3
  Gain3/1 -> Product/1
  Gain/1 -> Gain2/1
  Constant/1 -> Gain/1
  Cross Product2/1 -> Ps4/1
  Constant1/1 -> Dot Product1/2
  Gain2/1 -> Gain3/1

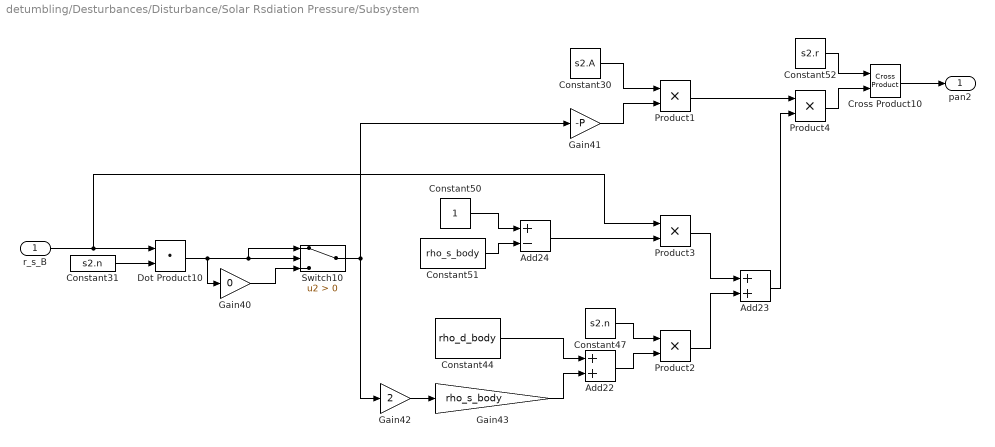
== system detumbling/Desturbances/Disturbance/Solar Rsdiation Pressure/Subsystem ==
  r_s_B : Inport
  Add22 : Sum
  Add23 : Sum
  Add24 : Sum  Inputs=+-
  Constant30 : Constant  Value=s2.A
  Constant31 : Constant  Value=s2.n
  Constant44 : Constant  Value=rho_d_body
  Constant47 : Constant  Value=s2.n
  Constant50 : Constant
  Constant51 : Constant  Value=rho_s_body
  Constant52 : Constant  Value=s2.r
  Cross Product10 : vrlib/Utilities/Cross Product
  Dot Product10 : DotProduct  OutDataTypeStr=Inherit: Inherit via internal rule
  Gain40 : Gain  Gain=0
  Gain41 : Gain  Gain=-P
  Gain42 : Gain  Gain=2
  Gain43 : Gain  Gain=rho_s_body
  Product{1..4} (4 alike) : Product
  Switch10 : Switch  Criteria=u2 > Threshold  SaturateOnIntegerOverflow=off  InputSameDT=off
  pan2 : Outport
  wires:
  Constant50/1 -> Add24/1
  Gain42/1 -> Gain43/1
  Cross Product10/1 -> pan2/1
  Gain43/1 -> Add22/2
  Constant52/1 -> Cross Product10/1
  Add22/1 -> Product2/2
  Gain41/1 -> Product1/2
  Gain40/1 -> Switch10/3
  Dot Product10/1 -> Gain40/1, Switch10/1, Switch10/2
  Product2/1 -> Add23/2
  Constant31/1 -> Dot Product10/2
  Constant51/1 -> Add24/2
  Add24/1 -> Product3/2
  Product3/1 -> Add23/1
  Constant44/1 -> Add22/1
  r_s_B/1 -> Product3/1, Dot Product10/1
  Product1/1 -> Product4/1
  Constant47/1 -> Product2/1
  Switch10/1 -> Gain41/1, Gain42/1
  Constant30/1 -> Product1/1
  Product4/1 -> Cross Product10/2
  Add23/1 -> Product4/2

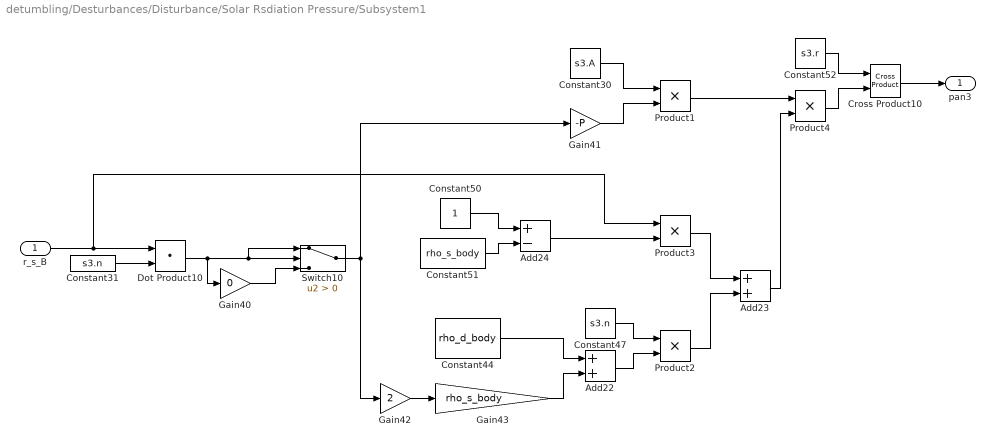
== system detumbling/Desturbances/Disturbance/Solar Rsdiation Pressure/Subsystem1 ==
  r_s_B : Inport
  Add22 : Sum
  Add23 : Sum
  Add24 : Sum  Inputs=+-
  Constant30 : Constant  Value=s3.A
  Constant31 : Constant  Value=s3.n
  Constant44 : Constant  Value=rho_d_body
  Constant47 : Constant  Value=s3.n
  Constant50 : Constant
  Constant51 : Constant  Value=rho_s_body
  Constant52 : Constant  Value=s3.r
  Cross Product10 : vrlib/Utilities/Cross Product
  Dot Product10 : DotProduct  OutDataTypeStr=Inherit: Inherit via internal rule
  Gain40 : Gain  Gain=0
  Gain41 : Gain  Gain=-P
  Gain42 : Gain  Gain=2
  Gain43 : Gain  Gain=rho_s_body
  Product{1..4} (4 alike) : Product
  Switch10 : Switch  Criteria=u2 > Threshold  SaturateOnIntegerOverflow=off  InputSameDT=off
  pan3 : Outport
  wires:
  Add23/1 -> Product4/2
  Product4/1 -> Cross Product10/2
  Constant30/1 -> Product1/1
  Switch10/1 -> Gain42/1, Gain41/1
  Constant47/1 -> Product2/1
  Product1/1 -> Product4/1
  r_s_B/1 -> Dot Product10/1, Product3/1
  Constant44/1 -> Add22/1
  Product3/1 -> Add23/1
  Add24/1 -> Product3/2
  Constant51/1 -> Add24/2
  Constant31/1 -> Dot Product10/2
  Product2/1 -> Add23/2
  Dot Product10/1 -> Switch10/2, Switch10/1, Gain40/1
  Gain40/1 -> Switch10/3
  Gain41/1 -> Product1/2
  Add22/1 -> Product2/2
  Constant52/1 -> Cross Product10/1
  Gain43/1 -> Add22/2
  Cross Product10/1 -> pan3/1
  Gain42/1 -> Gain43/1
  Constant50/1 -> Add24/1

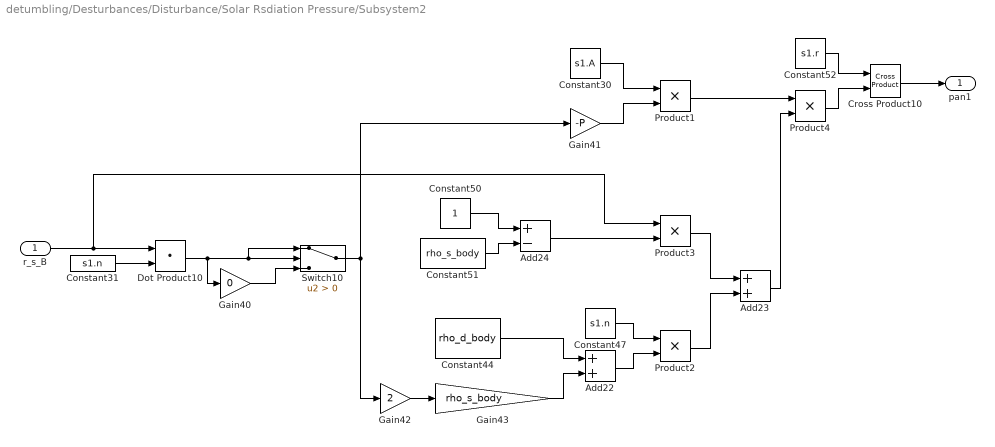
== system detumbling/Desturbances/Disturbance/Solar Rsdiation Pressure/Subsystem2 ==
  r_s_B : Inport
  Add22 : Sum
  Add23 : Sum
  Add24 : Sum  Inputs=+-
  Constant30 : Constant  Value=s1.A
  Constant31 : Constant  Value=s1.n
  Constant44 : Constant  Value=rho_d_body
  Constant47 : Constant  Value=s1.n
  Constant50 : Constant
  Constant51 : Constant  Value=rho_s_body
  Constant52 : Constant  Value=s1.r
  Cross Product10 : vrlib/Utilities/Cross Product
  Dot Product10 : DotProduct  OutDataTypeStr=Inherit: Inherit via internal rule
  Gain40 : Gain  Gain=0
  Gain41 : Gain  Gain=-P
  Gain42 : Gain  Gain=2
  Gain43 : Gain  Gain=rho_s_body
  Product{1..4} (4 alike) : Product
  Switch10 : Switch  Criteria=u2 > Threshold  SaturateOnIntegerOverflow=off  InputSameDT=off
  pan1 : Outport
  wires:
  Add23/1 -> Product4/2
  Product4/1 -> Cross Product10/2
  Constant30/1 -> Product1/1
  Switch10/1 -> Gain42/1, Gain41/1
  Constant47/1 -> Product2/1
  Product1/1 -> Product4/1
  r_s_B/1 -> Dot Product10/1, Product3/1
  Constant44/1 -> Add22/1
  Product3/1 -> Add23/1
  Add24/1 -> Product3/2
  Constant51/1 -> Add24/2
  Constant31/1 -> Dot Product10/2
  Product2/1 -> Add23/2
  Dot Product10/1 -> Switch10/2, Switch10/1, Gain40/1
  Gain40/1 -> Switch10/3
  Gain41/1 -> Product1/2
  Add22/1 -> Product2/2
  Constant52/1 -> Cross Product10/1
  Gain43/1 -> Add22/2
  Cross Product10/1 -> pan1/1
  Gain42/1 -> Gain43/1
  Constant50/1 -> Add24/1

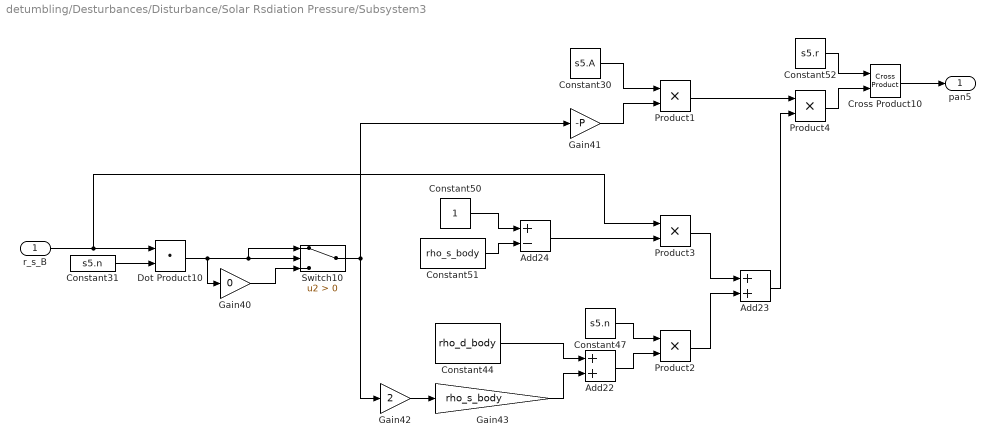
== system detumbling/Desturbances/Disturbance/Solar Rsdiation Pressure/Subsystem3 ==
  r_s_B : Inport
  Add22 : Sum
  Add23 : Sum
  Add24 : Sum  Inputs=+-
  Constant30 : Constant  Value=s5.A
  Constant31 : Constant  Value=s5.n
  Constant44 : Constant  Value=rho_d_body
  Constant47 : Constant  Value=s5.n
  Constant50 : Constant
  Constant51 : Constant  Value=rho_s_body
  Constant52 : Constant  Value=s5.r
  Cross Product10 : vrlib/Utilities/Cross Product
  Dot Product10 : DotProduct  OutDataTypeStr=Inherit: Inherit via internal rule
  Gain40 : Gain  Gain=0
  Gain41 : Gain  Gain=-P
  Gain42 : Gain  Gain=2
  Gain43 : Gain  Gain=rho_s_body
  Product{1..4} (4 alike) : Product
  Switch10 : Switch  Criteria=u2 > Threshold  SaturateOnIntegerOverflow=off  InputSameDT=off
  pan5 : Outport
  wires:
  Constant50/1 -> Add24/1
  Gain42/1 -> Gain43/1
  Cross Product10/1 -> pan5/1
  Gain43/1 -> Add22/2
  Constant52/1 -> Cross Product10/1
  Add22/1 -> Product2/2
  Gain41/1 -> Product1/2
  Gain40/1 -> Switch10/3
  Dot Product10/1 -> Gain40/1, Switch10/1, Switch10/2
  Product2/1 -> Add23/2
  Constant31/1 -> Dot Product10/2
  Constant51/1 -> Add24/2
  Add24/1 -> Product3/2
  Product3/1 -> Add23/1
  Constant44/1 -> Add22/1
  r_s_B/1 -> Product3/1, Dot Product10/1
  Product1/1 -> Product4/1
  Constant47/1 -> Product2/1
  Switch10/1 -> Gain41/1, Gain42/1
  Constant30/1 -> Product1/1
  Product4/1 -> Cross Product10/2
  Add23/1 -> Product4/2

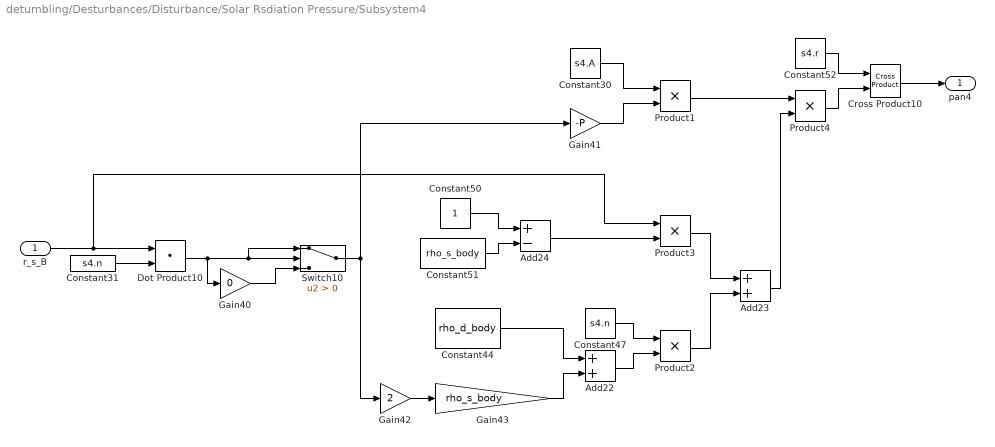
== system detumbling/Desturbances/Disturbance/Solar Rsdiation Pressure/Subsystem4 ==
  r_s_B : Inport
  Add22 : Sum
  Add23 : Sum
  Add24 : Sum  Inputs=+-
  Constant30 : Constant  Value=s4.A
  Constant31 : Constant  Value=s4.n
  Constant44 : Constant  Value=rho_d_body
  Constant47 : Constant  Value=s4.n
  Constant50 : Constant
  Constant51 : Constant  Value=rho_s_body
  Constant52 : Constant  Value=s4.r
  Cross Product10 : vrlib/Utilities/Cross Product
  Dot Product10 : DotProduct  OutDataTypeStr=Inherit: Inherit via internal rule
  Gain40 : Gain  Gain=0
  Gain41 : Gain  Gain=-P
  Gain42 : Gain  Gain=2
  Gain43 : Gain  Gain=rho_s_body
  Product{1..4} (4 alike) : Product
  Switch10 : Switch  Criteria=u2 > Threshold  SaturateOnIntegerOverflow=off  InputSameDT=off
  pan4 : Outport
  wires:
  Constant50/1 -> Add24/1
  Gain42/1 -> Gain43/1
  Cross Product10/1 -> pan4/1
  Gain43/1 -> Add22/2
  Constant52/1 -> Cross Product10/1
  Add22/1 -> Product2/2
  Gain41/1 -> Product1/2
  Gain40/1 -> Switch10/3
  Dot Product10/1 -> Gain40/1, Switch10/1, Switch10/2
  Product2/1 -> Add23/2
  Constant31/1 -> Dot Product10/2
  Constant51/1 -> Add24/2
  Add24/1 -> Product3/2
  Product3/1 -> Add23/1
  Constant44/1 -> Add22/1
  r_s_B/1 -> Product3/1, Dot Product10/1
  Product1/1 -> Product4/1
  Constant47/1 -> Product2/1
  Switch10/1 -> Gain41/1, Gain42/1
  Constant30/1 -> Product1/1
  Product4/1 -> Cross Product10/2
  Add23/1 -> Product4/2

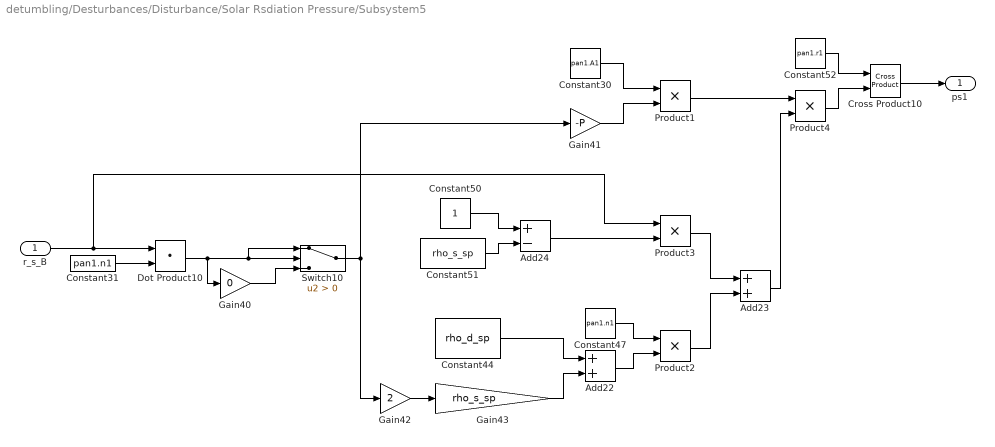
== system detumbling/Desturbances/Disturbance/Solar Rsdiation Pressure/Subsystem5 ==
  r_s_B : Inport
  Add22 : Sum
  Add23 : Sum
  Add24 : Sum  Inputs=+-
  Constant30 : Constant  Value=pan1.A1
  Constant31 : Constant  Value=pan1.n1
  Constant44 : Constant  Value=rho_d_sp
  Constant47 : Constant  Value=pan1.n1
  Constant50 : Constant
  Constant51 : Constant  Value=rho_s_sp
  Constant52 : Constant  Value=pan1.r1
  Cross Product10 : vrlib/Utilities/Cross Product
  Dot Product10 : DotProduct  OutDataTypeStr=Inherit: Inherit via internal rule
  Gain40 : Gain  Gain=0
  Gain41 : Gain  Gain=-P
  Gain42 : Gain  Gain=2
  Gain43 : Gain  Gain=rho_s_sp
  Product{1..4} (4 alike) : Product
  Switch10 : Switch  Criteria=u2 > Threshold  SaturateOnIntegerOverflow=off  InputSameDT=off
  ps1 : Outport
  wires:
  Add23/1 -> Product4/2
  Product4/1 -> Cross Product10/2
  Constant30/1 -> Product1/1
  Switch10/1 -> Gain42/1, Gain41/1
  Constant47/1 -> Product2/1
  Product1/1 -> Product4/1
  r_s_B/1 -> Dot Product10/1, Product3/1
  Constant44/1 -> Add22/1
  Product3/1 -> Add23/1
  Add24/1 -> Product3/2
  Constant51/1 -> Add24/2
  Constant31/1 -> Dot Product10/2
  Product2/1 -> Add23/2
  Dot Product10/1 -> Switch10/2, Switch10/1, Gain40/1
  Gain40/1 -> Switch10/3
  Gain41/1 -> Product1/2
  Add22/1 -> Product2/2
  Constant52/1 -> Cross Product10/1
  Gain43/1 -> Add22/2
  Cross Product10/1 -> ps1/1
  Gain42/1 -> Gain43/1
  Constant50/1 -> Add24/1

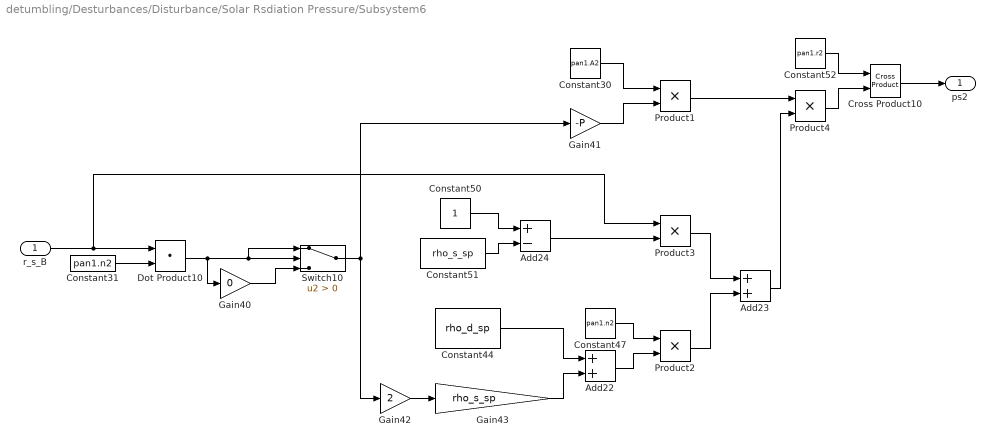
== system detumbling/Desturbances/Disturbance/Solar Rsdiation Pressure/Subsystem6 ==
  r_s_B : Inport
  Add22 : Sum
  Add23 : Sum
  Add24 : Sum  Inputs=+-
  Constant30 : Constant  Value=pan1.A2
  Constant31 : Constant  Value=pan1.n2
  Constant44 : Constant  Value=rho_d_sp
  Constant47 : Constant  Value=pan1.n2
  Constant50 : Constant
  Constant51 : Constant  Value=rho_s_sp
  Constant52 : Constant  Value=pan1.r2
  Cross Product10 : vrlib/Utilities/Cross Product
  Dot Product10 : DotProduct  OutDataTypeStr=Inherit: Inherit via internal rule
  Gain40 : Gain  Gain=0
  Gain41 : Gain  Gain=-P
  Gain42 : Gain  Gain=2
  Gain43 : Gain  Gain=rho_s_sp
  Product{1..4} (4 alike) : Product
  Switch10 : Switch  Criteria=u2 > Threshold  SaturateOnIntegerOverflow=off  InputSameDT=off
  ps2 : Outport
  wires:
  Constant50/1 -> Add24/1
  Gain42/1 -> Gain43/1
  Cross Product10/1 -> ps2/1
  Gain43/1 -> Add22/2
  Constant52/1 -> Cross Product10/1
  Add22/1 -> Product2/2
  Gain41/1 -> Product1/2
  Gain40/1 -> Switch10/3
  Dot Product10/1 -> Gain40/1, Switch10/1, Switch10/2
  Product2/1 -> Add23/2
  Constant31/1 -> Dot Product10/2
  Constant51/1 -> Add24/2
  Add24/1 -> Product3/2
  Product3/1 -> Add23/1
  Constant44/1 -> Add22/1
  r_s_B/1 -> Product3/1, Dot Product10/1
  Product1/1 -> Product4/1
  Constant47/1 -> Product2/1
  Switch10/1 -> Gain41/1, Gain42/1
  Constant30/1 -> Product1/1
  Product4/1 -> Cross Product10/2
  Add23/1 -> Product4/2

== system detumbling/Desturbances/Disturbance/Solar Rsdiation Pressure/Subsystem7 ==
  r_s_B : Inport
  Add22 : Sum
  Add23 : Sum
  Add24 : Sum  Inputs=+-
  Constant30 : Constant  Value=s6.A
  Constant31 : Constant  Value=s6.n
  Constant44 : Constant  Value=rho_d_body
  Constant47 : Constant  Value=s6.n
  Constant50 : Constant
  Constant51 : Constant  Value=rho_s_body
  Constant52 : Constant  Value=s6.r
  Cross Product10 : vrlib/Utilities/Cross Product
  Dot Product10 : DotProduct  OutDataTypeStr=Inherit: Inherit via internal rule
  Gain40 : Gain  Gain=0
  Gain41 : Gain  Gain=-P
  Gain42 : Gain  Gain=2
  Gain43 : Gain  Gain=rho_s_body
  Product{1..4} (4 alike) : Product
  Switch10 : Switch  Criteria=u2 > Threshold  SaturateOnIntegerOverflow=off  InputSameDT=off
  pan6 : Outport
  wires:
  Constant50/1 -> Add24/1
  Gain42/1 -> Gain43/1
  Cross Product10/1 -> pan6/1
  Gain43/1 -> Add22/2
  Constant52/1 -> Cross Product10/1
  Add22/1 -> Product2/2
  Gain41/1 -> Product1/2
  Gain40/1 -> Switch10/3
  Dot Product10/1 -> Gain40/1, Switch10/1, Switch10/2
  Product2/1 -> Add23/2
  Constant31/1 -> Dot Product10/2
  Constant51/1 -> Add24/2
  Add24/1 -> Product3/2
  Product3/1 -> Add23/1
  Constant44/1 -> Add22/1
  r_s_B/1 -> Product3/1, Dot Product10/1
  Product1/1 -> Product4/1
  Constant47/1 -> Product2/1
  Switch10/1 -> Gain41/1, Gain42/1
  Constant30/1 -> Product1/1
  Product4/1 -> Cross Product10/2
  Add23/1 -> Product4/2

== system detumbling/Desturbances/Disturbance/Solar Rsdiation Pressure/Subsystem8 ==
  r_s_B : Inport
  Add22 : Sum
  Add23 : Sum
  Add24 : Sum  Inputs=+-
  Constant30 : Constant  Value=pan2.A2
  Constant31 : Constant  Value=pan2.n2
  Constant44 : Constant  Value=rho_d_sp
  Constant47 : Constant  Value=pan2.n2
  Constant50 : Constant
  Constant51 : Constant  Value=rho_s_sp
  Constant52 : Constant  Value=pan2.r2
  Cross Product10 : vrlib/Utilities/Cross Product
  Dot Product10 : DotProduct  OutDataTypeStr=Inherit: Inherit via internal rule
  Gain40 : Gain  Gain=0
  Gain41 : Gain  Gain=-P
  Gain42 : Gain  Gain=2
  Gain43 : Gain  Gain=rho_s_sp
  Product{1..4} (4 alike) : Product
  Switch10 : Switch  Criteria=u2 > Threshold  SaturateOnIntegerOverflow=off  InputSameDT=off
  ps4 : Outport
  wires:
  Add23/1 -> Product4/2
  Product4/1 -> Cross Product10/2
  Constant30/1 -> Product1/1
  Switch10/1 -> Gain42/1, Gain41/1
  Constant47/1 -> Product2/1
  Product1/1 -> Product4/1
  r_s_B/1 -> Dot Product10/1, Product3/1
  Constant44/1 -> Add22/1
  Product3/1 -> Add23/1
  Add24/1 -> Product3/2
  Constant51/1 -> Add24/2
  Constant31/1 -> Dot Product10/2
  Product2/1 -> Add23/2
  Dot Product10/1 -> Switch10/2, Switch10/1, Gain40/1
  Gain40/1 -> Switch10/3
  Gain41/1 -> Product1/2
  Add22/1 -> Product2/2
  Constant52/1 -> Cross Product10/1
  Gain43/1 -> Add22/2
  Cross Product10/1 -> ps4/1
  Gain42/1 -> Gain43/1
  Constant50/1 -> Add24/1

== system detumbling/Desturbances/Disturbance/Solar Rsdiation Pressure/Subsystem9 ==
  r_s_B : Inport
  Add22 : Sum
  Add23 : Sum
  Add24 : Sum  Inputs=+-
  Constant30 : Constant  Value=pan2.A1
  Constant31 : Constant  Value=pan2.n1
  Constant44 : Constant  Value=rho_d_sp
  Constant47 : Constant  Value=pan2.n1
  Constant50 : Constant
  Constant51 : Constant  Value=rho_s_sp
  Constant52 : Constant  Value=pan2.r1
  Cross Product10 : vrlib/Utilities/Cross Product
  Dot Product10 : DotProduct  OutDataTypeStr=Inherit: Inherit via internal rule
  Gain40 : Gain  Gain=0
  Gain41 : Gain  Gain=-P
  Gain42 : Gain  Gain=2
  Gain43 : Gain  Gain=rho_s_sp
  Product{1..4} (4 alike) : Product
  Switch10 : Switch  Criteria=u2 > Threshold  SaturateOnIntegerOverflow=off  InputSameDT=off
  ps3 : Outport
  wires:
  Add23/1 -> Product4/2
  Product4/1 -> Cross Product10/2
  Constant30/1 -> Product1/1
  Switch10/1 -> Gain42/1, Gain41/1
  Constant47/1 -> Product2/1
  Product1/1 -> Product4/1
  r_s_B/1 -> Dot Product10/1, Product3/1
  Constant44/1 -> Add22/1
  Product3/1 -> Add23/1
  Add24/1 -> Product3/2
  Constant51/1 -> Add24/2
  Constant31/1 -> Dot Product10/2
  Product2/1 -> Add23/2
  Dot Product10/1 -> Switch10/2, Switch10/1, Gain40/1
  Gain40/1 -> Switch10/3
  Gain41/1 -> Product1/2
  Add22/1 -> Product2/2
  Constant52/1 -> Cross Product10/1
  Gain43/1 -> Add22/2
  Cross Product10/1 -> ps3/1
  Gain42/1 -> Gain43/1
  Constant50/1 -> Add24/1

== matlab function detumbling/Attitude Determination/Attitude Determination ==
  data: A_BN input; b_N input; A_BN_s output; accuracy1 input; A_eps1 input; r_N input; accuracy2 input; A_eps2 input
function A_BN_s = Wahba_solution(A_BN, b_N, accuracy1, A_eps1, r_N, accuracy2, A_eps2)

% Wahba's Problem: to solve the problem using a statistical method, at least 2 vector measurements 
% and the knowledge of relative precision of the sensors is needed to minimize
% the weighted error function.
% 
% INPUTS:
% A_BN [3x3] : DCM
% b_N_m [3x1] : vector measurement of first sensor [T]
% accuracy1 [1] : accuracy of the first sensor [deg]
% r_N_m [3x1] : vector measurement of second sensor [km]
% accuracy2 [1] : accuracy of the second sensor [deg]

v_N1 = b_N;
v_N2 = r_N;

s_B1 = A_eps1 * A_BN * v_N1;
s_B2 = A_eps2 * A_BN * v_N2;

precision1 = 1/deg2rad(accuracy1);
precision2 = 1/deg2rad(accuracy2);

% Weights normalization
alpha1 = precision1/(precision1+precision2);
alpha2 = precision2/(precision1+precision2);

% Solve for B
B = alpha1 * s_B1 * v_N1' + alpha2 * s_B2 * v_N2';

% Singular value decomposition
[U,~,V] = svd(B);
M = diag([1, 1, det(U)*det(V)]);
A_BN_s = U*M*V';

end
